simulink model "blockdemo"  (Simulink 6.3)
settings: Solver=VariableStepDiscrete  StartTime=0  StopTime=30  MaxStep=1  RelTol=1e-3
InitFcn:
  | %% DSPBuilder Start
  | alt_dspbuilder_update_model(bdroot)
  | %% DSPBuilder End
libraries: allblocks_alteradspbuilder2 x10
settings Model: Creator=cpurcell  LastModifiedBy=delphick
settings DebuggingCC: MultiTaskDSMMsg=error

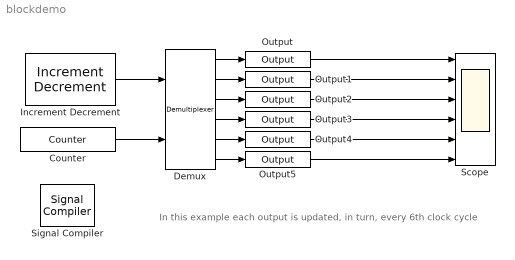
== system blockdemo ==
  note: In this example each output is updated, in turn, every 6th clock cycle
  Counter : allblocks_alteradspbuilder2/Counter  BusType=Unsigned Integer  bwl=3  bwr=0  use_modulo=on  modulo=6  SpecifyClock=off  direction=Increment  use_sload=off  use_sset=off  svalue=1  use_ena=off  use_sclr=off
  Demux : allblocks_alteradspbuilder2/Demultiplexer  numOutputs=6  use_ena=off  use_sclr=off
  Increment Decrement : allblocks_alteradspbuilder2/Increment Decrement  BusType=Unsigned Integer  bwl=6  bwr=8  SpecifyClock=off  clr_value=0  direction=Increment  phase_selection=1  use_ena=off  use_sclr=off
  Output : allblocks_alteradspbuilder2/Output  iofile=C:\workspace_clean\Documentation\DesignExamples\Tutorials\UnitBlocks\GateAndControl\Demultiplexer\tb_blockdemo\blockdemo_Output.capture  BusType=Inferred  bwl=8  bwr=0  PORTTYPE=Output
  Output1 : allblocks_alteradspbuilder2/Output  iofile=C:\workspace_clean\Documentation\DesignExamples\Tutorials\UnitBlocks\GateAndControl\Demultiplexer\tb_blockdemo\blockdemo_Output1.capture  BusType=Inferred  bwl=8  bwr=0  PORTTYPE=Output
  Output2 : allblocks_alteradspbuilder2/Output  iofile=C:\workspace_clean\Documentation\DesignExamples\Tutorials\UnitBlocks\GateAndControl\Demultiplexer\tb_blockdemo\blockdemo_Output2.capture  BusType=Inferred  bwl=8  bwr=0  PORTTYPE=Output
  Output3 : allblocks_alteradspbuilder2/Output  iofile=C:\workspace_clean\Documentation\DesignExamples\Tutorials\UnitBlocks\GateAndControl\Demultiplexer\tb_blockdemo\blockdemo_Output3.capture  BusType=Inferred  bwl=8  bwr=0  PORTTYPE=Output
  Output4 : allblocks_alteradspbuilder2/Output  iofile=C:\workspace_clean\Documentation\DesignExamples\Tutorials\UnitBlocks\GateAndControl\Demultiplexer\tb_blockdemo\blockdemo_Output4.capture  BusType=Inferred  bwl=8  bwr=0  PORTTYPE=Output
  Output5 : allblocks_alteradspbuilder2/Output  iofile=C:\workspace_clean\Documentation\DesignExamples\Tutorials\UnitBlocks\GateAndControl\Demultiplexer\tb_blockdemo\blockdemo_Output5.capture  BusType=Inferred  bwl=8  bwr=0  PORTTYPE=Output
  Scope : Scope  NumInputPorts=6
      settings: TimeRange=30  YMin=-1~-1~-1~-1~-1~-1  YMax=31~31~31~31~31~31
  Signal Compiler : allblocks_alteradspbuilder2/Signal Compiler  DeviceFamily=Stratix IV  DeviceName=AUTO  EnableSignalTap=off  SignalTapDepth=128  UseBoardBlock=off  StpUseDefaultClock=on  StpClock=clock
  wires:
  Counter/1 -> Demux/2
  Increment Decrement/1 -> Demux/1
  Demux/1 -> Output/1
  Demux/2 -> Output1/1
  Demux/3 -> Output2/1
  Demux/4 -> Output3/1
  Demux/5 -> Output4/1
  Demux/6 -> Output5/1
  Output/1 -> Scope/1
  Output1/1 -> Scope/2
  Output2/1 -> Scope/3
  Output3/1 -> Scope/4
  Output4/1 -> Scope/5
  Output5/1 -> Scope/6
